simulink model "ZC_infinis"  (R2016b)
settings: Solver=VariableStepAuto  StartTime=0.0  StopTime=10.0  RelTol=1e-3
settings Model: Creator=live  LastModifiedBy=live

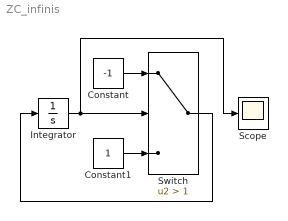
== system ZC_infinis ==
  Constant : Constant  Value=-1
  Constant1 : Constant
  Integrator : Integrator
  Scope : Scope
  Switch : Switch  Criteria=u2 > Threshold  Threshold=1
  wires:
  Constant/1 -> Switch/1
  Constant1/1 -> Switch/3
  Integrator/1 -> Scope/1, Switch/2
  Switch/1 -> Integrator/1
